simulink model "Chapter_4_Section_3_Model"  (R2017a)
settings: Solver=ode4  StartTime=0.0  StopTime=200  FixedStep=stp_sz  MaxStep=.0001  MinStep=.00005  RelTol=1e-7  AbsTol=1e-7  EnableMultiTasking=on
InitFcn:
  | load Chapter_4_Section_3
  | warning off
StopFcn:
  | save data.mat u_simulation v_simulation psi_simulation r_simulation npr_user_provided npr_achievable alpha_user_provided alpha_achievable stp_sz
  | clear all
  | load('data.mat')
  | delete('data.mat')
values from neighbouring files (symbols this model uses):
  A_disk = 13.2025431267    [Chapter_4_Section_3.mat]
  a_r11 = [-0.000865667853776 -0.901318756108 0.00874486630837 -0.00765974060328 0.00955717632387 0.00641813989061 -0.011076069832 0.00201248118094 -0.00501952733262 0.00315605586996 -0.00210851076531 0.0148609220099 ... (324 elements, 18x18)]    [Chapter_4_Section_3.mat]
  a_r13 = [-0.0294995912119 -4.91037219533 -0.00332739568397 0.0888755061346 -0.00681796875441 0.183812407485 0.0112008036726 0.10429312155 -0.0251601482875 -0.228675692165 0.00453476042855 0.0594697753606 ... (169 elements, 13x13)]    [Chapter_4_Section_3.mat]
  a_r15 = [-0.00127786555898 0.776225741104 -0.00474776997752 -0.00131066749835 0.0137520402687 -0.00211384579247 8.8019955143e-05 -0.00028996241197 -0.00129826872567 -0.0202543144732 0.0030370404199 -0.00453425604591 ... (169 elements, 13x13)]    [Chapter_4_Section_3.mat]
  a_r22 = [-0.000797108949019 -1.01015556887 0.00406573750109 -0.00111578544774 0.00423859757219 -0.00799128279013 0.00569024815652 -0.0167562674532 0.00334935655618 -0.000712432292804 0.00154242142086 0.00240437743229 ... (169 elements, 13x13)]    [Chapter_4_Section_3.mat]
  a_r24 = [-0.000686927823555 -0.95665602689 0.00244839898375 0.00145613314595 -0.00607023426216 0.0163996841317 0.00152022458075 -0.000736874734971 -0.00294919321651 -0.000761800577268 -0.00251686123035 -0.00197732815976 ... (169 elements, 13x13)]    [Chapter_4_Section_3.mat]
  a_r26 = [-0.194397873228 1.89810259721 -0.0873186628061 -0.241231729519 0.281206161775 -0.16994038615 -0.116565511469 -0.0496572593209 0.0216084469732 0.0912933167406 0.0299797727001 0.0314987707028 ... (169 elements, 13x13)]    [Chapter_4_Section_3.mat]
  a_r31 = [-0.00489112559449 -3.89960530455 -0.0361162658575 0.0265931197764 0.0034376033088 0.000316401308368 -0.0243996243526 0.0792200139858 -0.023187698537 -0.0726743997029 0.00400632061963 -0.0350516560041 ... (169 elements, 13x13)]    [Chapter_4_Section_3.mat]
  a_r33 = [-0.601431448276 0.50360246711 0.500115950342 -0.0452293844892 -0.0181314142185 -0.0323524621531 0.0355826051968 0.0329239610677 0.0940919952313 0.0566642992805 -0.0379178935102 0.0254835488846 ... (169 elements, 13x13)]    [Chapter_4_Section_3.mat]
  a_r35 = [-0.861988746714 -0.582511154549 0.34264856173 -0.0655310417272 -0.417167685168 0.183176698588 -0.473887691644 -0.225677727522 -0.133571139717 -0.218168843707 0.0850592077583 -0.0257492082836 ... (169 elements, 13x13)]    [Chapter_4_Section_3.mat]
  a_r42 = [-0.000411079312172 -0.966350953459 0.00419936729713 0.00358740198521 -0.00356571428733 -0.00958951498266 -0.00230062261745 -3.48708248632e-05 -0.00350313209064 -0.00772126326768 -0.0011918234528 -0.00149424537901 ... (169 elements, 13x13)]    [Chapter_4_Section_3.mat]
  a_r44 = [-0.000156115728087 -0.944139704333 -0.00242185567679 0.00620214191605 0.00232565005277 -0.00625050722164 0.00126021167241 -0.000681873506535 0.0011931592381 -0.00289361611357 -0.00138182415247 -0.00252837386868 ... (169 elements, 13x13)]    [Chapter_4_Section_3.mat]
  a_r46 = [-0.000218462457517 1.89677852742 0.00896242354968 -0.00290259500747 0.00225128874867 0.00254539590487 0.00120681433209 0.00261900930035 0.00149629742842 0.000796832004109 0.00199591847947 0.00352664402036 ... (169 elements, 13x13)]    [Chapter_4_Section_3.mat]
  a_r51 = [-0.0010898880101 0.776080724329 0.000225388678941 0.00375234840616 -0.00838297691459 -0.00447310416982 -0.0119510882322 -0.00692765468718 0.00227273345413 -0.0063592610709 0.000914007544175 0.00943534814934 ... (169 elements, 13x13)]    [Chapter_4_Section_3.mat]
  a_r53 = [-0.83377539904 0.569677058563 0.434285019976 0.157205409215 -0.397195569542 -0.255164078245 -0.141246880777 0.177451291189 -0.182828550566 0.0648162508754 0.244251292681 0.160100487197 ... (169 elements, 13x13)]    [Chapter_4_Section_3.mat]
  a_r55 = [-0.000352406331634 0.764343029796 0.00339830320259 -0.000678251137483 -0.00243783779313 -0.00215979913278 0.00196909451093 -0.00577428819561 -0.00349811892924 -0.00488920883323 0.00112064970343 0.000774855197444 ... (169 elements, 13x13)]    [Chapter_4_Section_3.mat]
  a_r62 = [-0.546519039316 -1.22303009993 0.393735845548 -0.120016588191 0.38151861373 -0.213578592342 -0.602267954372 -0.105716444149 -0.153151371839 -0.163939447448 -0.555540353196 0.0685401630267 ... (169 elements, 13x13)]    [Chapter_4_Section_3.mat]
  a_r64 = [-0.0406191100017 -5.18251105957 -0.115497941507 -0.0935821370219 0.180972853448 -0.0201998949456 -0.0698170640352 -0.0736823539521 -0.034828919888 0.0876659960431 -0.0419335596239 -0.0240984963396 ... (169 elements, 13x13)]    [Chapter_4_Section_3.mat]
  a_r66 = [-0.00276803466684 1.11530008029 0.0229779449181 0.0262185319857 0.00628472844795 0.000156167369042 -0.00250093023805 -0.0114435042874 -0.00826774415326 -0.00991601759993 -0.00812142854996 0.0148245002111 ... (169 elements, 13x13)]    [Chapter_4_Section_3.mat]
  A_rudder = 6    [Chapter_4_Section_3.mat]
  alpha_max = 0.392699081699    [Chapter_4_Section_3.mat]
  b_r11 = [-1.91804272115 -67.7547902158 12.3212653748 -6.25011871643 13.082442224 5.48501776184 -10.1596546398 2.56004852009 -4.74360113798 3.95981895348 -2.02856412397 18.3264246889 ... (18 elements, 18x1)]    [Chapter_4_Section_3.mat]
  b_r13 = [9.68113335046 8.54720242819 0.883931047444 -5.56576078332 1.72641800243 -13.8756826027 -2.702777864 -9.4621991361 5.92943514782 22.6516835054 -1.0074598861 -6.31102592982 ... (13 elements, 13x1)]    [Chapter_4_Section_3.mat]
  b_r22 = [-8.230214728 -263.156134326 24.2327808151 -4.87921448873 19.1715641288 -45.8768653263 26.6325387064 -91.9399975548 16.6663243552 -3.80929112747 7.68030110892 12.8381492859 ... (13 elements, 13x1)]    [Chapter_4_Section_3.mat]
  b_r24 = [20.6689502907 674.321335078 -41.3637763247 -19.2444203625 82.0775505272 -259.897803047 -22.2545830602 11.3827604156 43.2189922355 11.7516897475 36.9394390446 30.4503929007 ... (13 elements, 13x1)]    [Chapter_4_Section_3.mat]
  b_r26 = [206.794755218 -62.242559329 24.5666904254 184.158146246 -103.419961827 115.160111337 76.4499795128 20.3457431208 -13.1704465249 -41.5730935141 -18.1334448714 -14.4641153742 ... (13 elements, 13x1)]    [Chapter_4_Section_3.mat]
  b_r31 = [3.76230189948 5.16928151238 2.64945725635 -18.4251953385 -2.0625905672 -0.18887543415 4.20433084471 -14.07893046 13.0563354882 16.4007691754 -2.13849071942 8.28528512456 ... (13 elements, 13x1)]    [Chapter_4_Section_3.mat]
  b_r33 = [-425.265727934 16.4952177922 163.76327445 -15.539902078 -6.59006558263 -11.1862310226 12.8543123126 11.4260264426 33.8206936715 19.7626944669 -13.5783728882 8.91023495161 ... (13 elements, 13x1)]    [Chapter_4_Section_3.mat]
  b_r35 = [955.467057384 23.8174564739 -126.402446683 48.3788727465 168.435579445 -128.161344325 216.24493699 142.979450788 65.1193355403 134.911935543 -50.7648858119 13.1799100865 ... (13 elements, 13x1)]    [Chapter_4_Section_3.mat]
  b_r42 = [15.9360311823 665.959154186 -98.5777560157 -55.5400651809 61.9220987195 200.312325561 47.5124103398 0.631683490985 64.1219861023 155.750535985 22.3985447876 29.803792586 ... (13 elements, 13x1)]    [Chapter_4_Section_3.mat]
  b_r44 = [-27.1891200017 -1761.50772747 -283.391471232 367.311489951 182.522124626 -579.755911925 104.353356772 -62.2376848714 99.3185259533 -260.784153955 -116.536414334 -226.454300618 ... (13 elements, 13x1)]    [Chapter_4_Section_3.mat]
  b_r46 = [-26.6906838426 431.487773123 657.709356633 -144.976364483 114.646575538 180.775978583 85.0953284375 135.592940904 78.9082960716 55.2973047721 106.740201988 241.432567993 ... (13 elements, 13x1)]    [Chapter_4_Section_3.mat]
  b_r51 = [-27.9768378982 741.05041888 2.33758926296 57.3995096963 -127.005620965 -47.2947833409 -133.876425682 -98.5907202753 26.0445243962 -88.3721242204 10.7680008324 130.122749963 ... (13 elements, 13x1)]    [Chapter_4_Section_3.mat]
  b_r53 = [949.455593416 -23.2452293814 -157.318364745 -121.412853107 173.067821874 177.10214052 64.7164189373 -120.452255472 86.0623964314 -43.0643550932 -116.39314584 -105.497696438 ... (13 elements, 13x1)]    [Chapter_4_Section_3.mat]
  b_r55 = [-217.127382907 9506.32343029 1148.82922273 -188.742556573 -694.43970838 -709.996440288 566.872400877 -1877.38940059 -1026.37679575 -1566.80129668 332.089563592 247.692614281 ... (13 elements, 13x1)]    [Chapter_4_Section_3.mat]
  b_r62 = [259.61149635 16.5485296799 -38.0095496792 45.1883806678 -40.3107166739 78.3455844965 73.5107367495 37.0054960802 51.6709447748 22.7410486275 84.4875008959 -21.9559289205 ... (13 elements, 13x1)]    [Chapter_4_Section_3.mat]
  b_r64 = [156.539833252 187.686482031 376.820920142 59.4312894666 -548.902692032 17.0176436095 70.7484878223 206.821047291 37.1716677759 -243.032149857 114.824775027 27.0037475025 ... (13 elements, 13x1)]    [Chapter_4_Section_3.mat]
  b_r66 = [-314.266256408 5285.46587095 1093.01941502 1627.30071258 387.633965073 8.0986510694 -130.443621448 -701.343286032 -436.49966457 -600.0481003 -433.735518303 884.367320612 ... (13 elements, 13x1)]    [Chapter_4_Section_3.mat]
  bettas_CQ = [0 5.39 17.77 34.97 50.79 58.7 64.55 68.33 73.49 85.2 93.11 102.75 ... (40 elements, 1x40)]    [Chapter_4_Section_3.mat]    (also in looking_up_n.m = [0 5.39 17.77 34.97 50.79 58.7 64.55 68.33 73.49 85.2 93.11 )
  bettas_CT = [0 5.37 16.73 33.6 44.63 60.82 73.22 80.46 86.3 92.15 100.41 110.74 ... (52 elements, 1x52)]    [Chapter_4_Section_3.mat]    (also in looking_up_n.m = [0 5.37 16.73 33.6 44.63 60.82 73.22 80.46 86.3 92.15 100.41)
  c_r11 = [1.91804272142 -67.7547902158 -12.3212653748 -6.25011871643 -13.082442224 5.48501776185 -10.1596546398 -2.56004852009 -4.74360113798 -3.95981895348 -2.02856412396 -18.3264246889 ... (18 elements, 1x18)]    [Chapter_4_Section_3.mat]
  c_r13 = [9.68113335045 -8.54720242824 0.883931047418 5.56576078332 1.72641800244 13.8756826027 -2.702777864 9.4621991361 5.92943514781 -22.6516835054 -1.0074598861 6.31102592982 ... (13 elements, 1x13)]    [Chapter_4_Section_3.mat]
  c_r22 = [8.23021472807 -263.156134326 -24.2327808151 -4.87921448871 19.1715641288 45.8768653263 26.6325387064 91.9399975548 16.6663243552 3.80929112749 7.68030110892 -12.8381492859 ... (13 elements, 1x13)]    [Chapter_4_Section_3.mat]
  c_r24 = [20.6689502903 -674.321335078 -41.3637763247 19.2444203625 -82.0775505271 -259.897803047 22.2545830602 11.3827604156 -43.2189922355 11.7516897475 -36.9394390446 30.4503929007 ... (13 elements, 1x13)]    [Chapter_4_Section_3.mat]
  c_r26 = [-206.794755218 -62.2425593289 24.5666904254 -184.158146246 -103.419961827 -115.160111337 -76.4499795128 20.3457431209 13.1704465249 -41.5730935141 18.1334448714 -14.4641153742 ... (13 elements, 1x13)]    [Chapter_4_Section_3.mat]
  c_r31 = [3.76230189951 -5.16928151238 -2.64945725636 -18.4251953385 -2.0625905672 -0.188875434257 -4.2043308447 14.07893046 13.0563354882 -16.4007691754 -2.13849071943 -8.28528512456 ... (13 elements, 1x13)]    [Chapter_4_Section_3.mat]
  c_r33 = [-425.265727934 -16.4952177923 -163.76327445 15.539902078 -6.5900655826 11.1862310226 12.8543123126 -11.4260264426 33.8206936715 -19.7626944669 -13.5783728882 -8.91023495161 ... (13 elements, 1x13)]    [Chapter_4_Section_3.mat]
  c_r35 = [-955.467057384 23.8174564746 -126.402446683 -48.3788727464 168.435579445 128.161344325 216.24493699 -142.979450788 65.1193355403 -134.911935543 50.7648858119 13.1799100865 ... (13 elements, 1x13)]    [Chapter_4_Section_3.mat]
  c_r42 = [15.9360311824 -665.959154186 -98.5777560157 55.5400651809 -61.9220987195 200.312325561 47.5124103398 -0.631683490192 -64.1219861023 155.750535985 -22.3985447876 29.803792586 ... (13 elements, 1x13)]    [Chapter_4_Section_3.mat]
  c_r44 = [27.189120009 -1761.50772747 283.391471232 367.311489951 182.522124626 579.755911925 104.353356772 62.2376848713 99.3185259533 260.784153955 -116.536414334 226.454300618 ... (13 elements, 1x13)]    [Chapter_4_Section_3.mat]
  c_r46 = [26.6906838375 431.487773123 -657.709356633 -144.976364484 114.646575538 -180.775978583 -85.0953284373 135.592940904 78.9082960717 -55.297304772 106.740201988 -241.432567993 ... (13 elements, 1x13)]    [Chapter_4_Section_3.mat]
  c_r51 = [27.9768378982 741.05041888 2.33758926325 -57.3995096963 127.005620965 -47.2947833409 -133.876425682 98.5907202753 26.0445243962 88.3721242204 10.7680008324 -130.122749963 ... (13 elements, 1x13)]    [Chapter_4_Section_3.mat]
  c_r53 = [-949.455593416 -23.2452293814 -157.318364745 121.412853107 173.067821874 -177.10214052 64.7164189374 120.452255472 86.0623964314 43.0643550932 -116.39314584 105.497696438 ... (13 elements, 1x13)]    [Chapter_4_Section_3.mat]
  c_r55 = [217.12738291 9506.32343029 -1148.82922273 -188.742556576 -694.43970838 709.996440288 566.872400876 1877.38940059 -1026.37679575 1566.80129668 332.089563594 -247.69261428 ... (13 elements, 1x13)]    [Chapter_4_Section_3.mat]
  c_r62 = [-259.61149635 16.5485296799 -38.0095496792 -45.1883806678 -40.3107166739 -78.3455844965 73.5107367495 -37.0054960802 -51.6709447748 22.7410486275 84.4875008959 21.9559289205 ... (13 elements, 1x13)]    [Chapter_4_Section_3.mat]
  c_r64 = [-156.539833251 187.686482031 -376.820920142 59.4312894666 548.902692032 17.0176436097 70.7484878223 -206.82104729 37.1716677758 243.032149857 -114.824775027 27.0037475025 ... (13 elements, 1x13)]    [Chapter_4_Section_3.mat]
  c_r66 = [314.266256408 5285.46587095 1093.01941502 -1627.30071258 -387.633965073 8.09865107118 -130.443621448 701.343286032 -436.49966457 600.0481003 -433.735518303 -884.367320612 ... (13 elements, 1x13)]    [Chapter_4_Section_3.mat]
  CQs = [0.008 0.007 -0.002 -0.018 -0.037 -0.049 -0.06 -0.065 -0.068 -0.059 -0.057 -0.059 ... (40 elements, 1x40)]    [Chapter_4_Section_3.mat]    (also in looking_up_n.m = -0.1.*[-0.08 -0.07 0.02 0.18 0.37 0.49 0.6 0.65 0.68 0.59 0.)
  CTs = [0.32 0.29 0.19 0.01 -0.16 -0.46 -0.7 -0.77 -0.7 -0.63 -0.63 -0.69 ... (52 elements, 1x52)]    [Chapter_4_Section_3.mat]    (also in looking_up_n.m = [0.32 0.29 0.19 0.01 -0.16 -0.46 -0.7 -0.77 -0.7 -0.63 -0.63)
  d_r11 = 95.5285227708    [Chapter_4_Section_3.mat]
  d_r13 = -14.1628545989    [Chapter_4_Section_3.mat]
  d_r22 = 1468.51041279    [Chapter_4_Section_3.mat]
  d_r24 = -9785.77027698    [Chapter_4_Section_3.mat]
  d_r26 = -1700.92421833    [Chapter_4_Section_3.mat]
  d_r31 = -0.95522945761    [Chapter_4_Section_3.mat]
  d_r33 = 3827.81220596    [Chapter_4_Section_3.mat]
  d_r35 = -19539.5268707    [Chapter_4_Section_3.mat]
  d_r42 = -9418.04264727    [Chapter_4_Section_3.mat]
  d_r44 = 68252.1479072    [Chapter_4_Section_3.mat]
  d_r46 = -10162.1377852    [Chapter_4_Section_3.mat]
  d_r51 = 12054.4514237    [Chapter_4_Section_3.mat]
  d_r53 = -19539.5038011    [Chapter_4_Section_3.mat]
  d_r55 = 1991036.95813    [Chapter_4_Section_3.mat]
  d_r62 = -1405.47636444    [Chapter_4_Section_3.mat]
  d_r64 = -12342.2523681    [Chapter_4_Section_3.mat]
  d_r66 = 610786.440495    [Chapter_4_Section_3.mat]
  DEN = 5.34671106464e+28    [Chapter_4_Section_3.mat]
  dist_LOS = [-50 -49 -48 -47 -46 -45 -44 -43 -42 -41 -40 -39 ... (1051 elements, 1x1051)]    [Chapter_4_Section_3.mat]
  Dpr = 4.1    [Chapter_4_Section_3.mat]    (also in looking_up_n.m = u(4))
  Dw = 0.110526315789    [Chapter_4_Section_3.mat]
  dx = 10    [Chapter_4_Section_3.mat]
  dxr = 48.75    [Chapter_4_Section_3.mat]
  dy = 2    [Chapter_4_Section_3.mat]
  dz = 0.8    [Chapter_4_Section_3.mat]
  dzr = 0.514285714286    [Chapter_4_Section_3.mat]
  g = 10    [Chapter_4_Section_3.mat]
  gravity = 10    [Chapter_4_Section_3.mat]
  INDEX = [1 2 3 4 5 6 7 8 9]    [Chapter_4_Section_3.mat]
  Ix = 724554000    [Chapter_4_Section_3.mat]
  Iy = 4528460000    [Chapter_4_Section_3.mat]
  Iz = 4528460000    [Chapter_4_Section_3.mat]
  k_wave = [0.0157865285852 0.0224311321394 0.0345394916241 0.0578593033576 0.0778685019714 0.0983501894009 0.10403521245 0.134043066308 0.155236404606 0.203205074918 0.220032771713 0.262178651673 ... (20 elements, 1x20)]    [Chapter_4_Section_3.mat]
  Last_Pt_Accuracy = 30    [Chapter_4_Section_3.mat]
  LBP = 100    [Chapter_4_Section_3.mat]
  m = 7264000    [Chapter_4_Section_3.mat]
  phase = [4.61787442739 6.09845039199 5.44708367148 0.54182753101 2.30238916367 2.31974450279 4.30416083443 3.75697809799 4.95971993271 2.31003141527 1.29451121971 0.54454197722 ... (20 elements, 1x20)]    [Chapter_4_Section_3.mat]
  phi_0 = 0    [Chapter_4_Section_3.mat]
  psi_0 = 0    [Chapter_4_Section_3.mat]
  R_convrg = 220    [Chapter_4_Section_3.mat]
  radius_LOS = [166.575605377 166.637026665 166.698699321 166.760625342 166.82280675 166.885245588 166.947943925 167.010903854 167.074127493 167.137616985 167.201374499 167.265402228 ... (1051 elements, 1x1051)]    [Chapter_4_Section_3.mat]
  raw = 1000    [Chapter_4_Section_3.mat]    (also in looking_up_n.m = u(3))
  s = 0.15    [Chapter_4_Section_3.mat]
  S11 = 5.22457985714e+28    [Chapter_4_Section_3.mat]
  S13 = 3.79917831589e+26    [Chapter_4_Section_3.mat]
  S15 = -4.97006200608e+19    [Chapter_4_Section_3.mat]
  S22 = 4.58630932583e+28    [Chapter_4_Section_3.mat]
  S24 = 9.38800137353e+19    [Chapter_4_Section_3.mat]
  S26 = 1.30387886946e+18    [Chapter_4_Section_3.mat]
  S31 = 3.83422033136e+26    [Chapter_4_Section_3.mat]
  S33 = 1.77296018417e+28    [Chapter_4_Section_3.mat]
  S35 = 2.44593333777e+19    [Chapter_4_Section_3.mat]
  S42 = 8.93369784557e+19    [Chapter_4_Section_3.mat]
  S44 = 7.37931315974e+19    [Chapter_4_Section_3.mat]
  S46 = 27990784014.6    [Chapter_4_Section_3.mat]
  S51 = -4.98658939538e+19    [Chapter_4_Section_3.mat]
  S53 = 2.45188465874e+19    [Chapter_4_Section_3.mat]
  S55 = 1.18069051188e+19    [Chapter_4_Section_3.mat]
  S62 = 1.30580221388e+18    [Chapter_4_Section_3.mat]
  S64 = 23535167243.9    [Chapter_4_Section_3.mat]
  S66 = 1.18069078235e+19    [Chapter_4_Section_3.mat]
  ... (+18 more)
undefined symbols (not defined in the file or in its folder): magnitude
libraries: simulink x9
(part 1 of 6)
CloseFcn:
  | rtwprivate ssgencode ModelCloseRequest editted_june25_edit_radius
settings Model: Creator=Nassim Khaled  LastModifiedBy=nassi
settings SolverCC: MaxConsecutiveMinStep=100
settings DataIOCC: Decimation=100  LimitDataPoints=on  MaxDataPoints=2500000  SaveFormat=Array  SignalLoggingSaveFormat=ModelDataLogs  SaveOutput=off  SignalLogging=off  SaveTime=off  OutputOption=SpecifiedOutputTimes  OutputTimes=0:.2:200
settings OptimizationCC: BooleanDataType=off  OptimizeBlockIOStorage=off  BufferReuse=off  GlobalBufferReuse=off  ExpressionFolding=off  ExpressionDepthLimit=2147483647  LocalBlockOutputs=off  InitFltsAndDblsToZero=on  LifeSpan=inf
settings DebuggingCC: ConsistencyChecking=warning  SaveWithParameterizedLinksMsg=none  UnderspecifiedInitializationDetection=Classic  MergeDetectMultiDrivingBlocksExec=none  SignalResolutionControl=TryResolveAllWithWarning  MaxConsecutiveZCsMsg=warning  SolverPrmCheckMsg=warning  MultiTaskDSMMsg=warning  MultiTaskCondExecSysMsg=warning  MultiTaskRateTransMsg=warning  FcnCallInpInsideContextMsg=warning  ModelReferenceExtraNoncontSigs=warning  StateNameClashWarn=warning  SFUnexpectedBacktrackingDiag=warning  SFNoUnconditionalDefaultTransitionDiag=warning  SFExecutionAtInitializationDiag=none
settings HardwareCC: ProdBitPerPointer=32  ProdBitPerSizeT=32  ProdBitPerPtrDiffT=32  ProdLargestAtomicFloat=None  ProdIntDivRoundTo=Undefined  ProdEndianess=Unspecified  ProdWordSize=32  ProdHWDeviceType=32-bit Generic  TargetBitPerPointer=64  TargetBitPerSizeT=64  TargetBitPerPtrDiffT=64  TargetLongLongMode=on  TargetIntDivRoundTo=Zero  TargetEndianess=LittleEndian  TargetWordSize=64  TargetHWDeviceType=MATLAB Host  ProdEqTarget=off
settings ModelReferenceCC: PropagateSignalLabelsOutOfModel=off
settings SFSimCC: SimParseCustomCode=off
settings RTWCC: SystemTargetFile=rsim.tlc  TemplateMakefile=rsim_default_tmf  Description=Rapid Simulation Target
settings ConfigComp: CovMetricSettings=dw  CovHtmlReporting=on  CovSaveCumulativeToWorkspaceVar=on  CovSaveSingleToWorkspaceVar=on  CovExternalEMLEnable=off

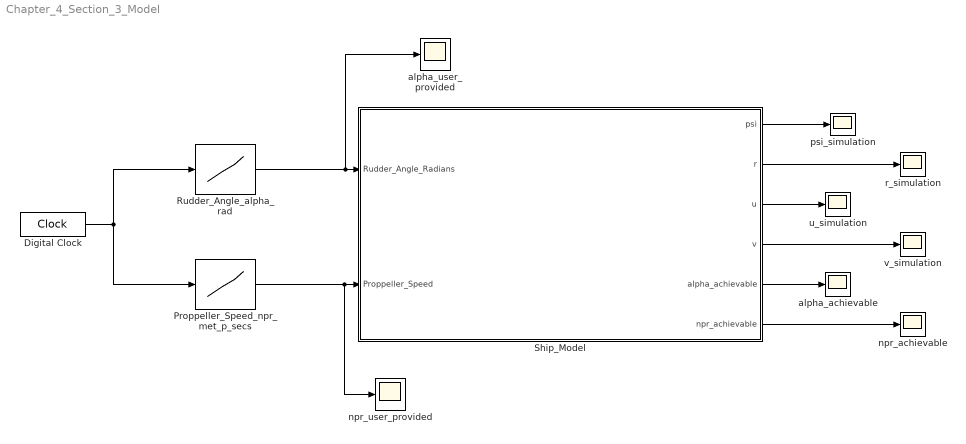
== system Chapter_4_Section_3_Model ==
  Digital Clock : DigitalClock  SampleTime=stp_sz
  Proppeller_Speed_npr_met_p_secs : Lookup_n-D  NumberOfTableDimensions=1  BreakpointsForDimension1=[0 75 100.2 150]  Table=[10 10 15 15 ]  InternalRulePriority=Speed  RndMeth=Simplest  InputSameDT=on
  Rudder_Angle_alpha_rad : Lookup_n-D  NumberOfTableDimensions=1  BreakpointsForDimension1="[0 25  42.5 150]"  Table=[0 0 0.1745 0.1745]  InternalRulePriority=Speed  RndMeth=Simplest  InputSameDT=on
  Ship_Model : Subsystem
  alpha_achievable : Scope
  alpha_user_provided : Scope
  npr_achievable : Scope
  npr_user_provided : Scope
  psi_simulation : Scope
  r_simulation : Scope
  u_simulation : Scope
  v_simulation : Scope
  wires:
  Proppeller_Speed_npr_met_p_secs/1 -> Ship_Model/2(Proppeller_Speed), npr_user_provided/1
  Rudder_Angle_alpha_rad/1 -> alpha_user_provided/1, Ship_Model/1(Rudder_Angle_Radians)
  Ship_Model/1(psi) -> psi_simulation/1
  Ship_Model/2(r) -> r_simulation/1
  Ship_Model/3(u) -> u_simulation/1
  Ship_Model/4(v) -> v_simulation/1
  Digital Clock/1 -> Rudder_Angle_alpha_rad/1, Proppeller_Speed_npr_met_p_secs/1
  Ship_Model/5(alpha_achievable) -> alpha_achievable/1
  Ship_Model/6(npr_achievable) -> npr_achievable/1

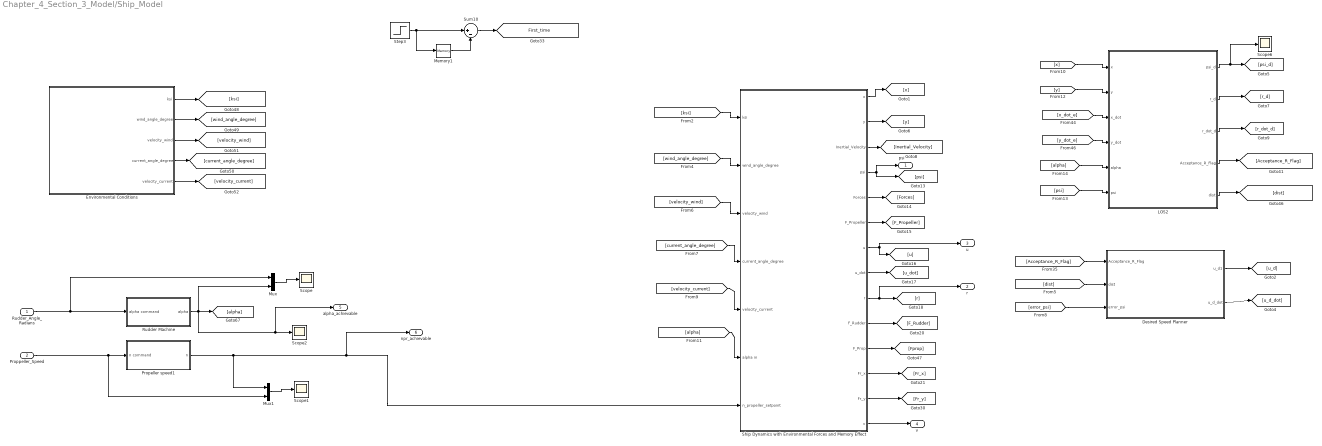
== system Chapter_4_Section_3_Model/Ship_Model ==
  Rudder_Angle_Radians : Inport
  Proppeller_Speed : Inport  Port=2
  Desired Speed Planner : Subsystem
  Environmental Conditions : Subsystem
  LOS2 : Subsystem
  Memory1 : Memory  InheritSampleTime=on
  Mux : Mux  Inputs=2
  Mux1 : Mux  Inputs=2
  Propeller speed1 : Subsystem
  Rudder Machine : Subsystem
  Scope{,1..2,6} (4 alike) : Scope
  Ship Dynamics with Environmental Forces and Memory Effect : Subsystem
  Step3 : Step  Time=0  SampleTime=0
  Sum10 : Sum  Inputs=|+-
  psi : Outport
  r : Outport  Port=2
  u : Outport  Port=3
  v : Outport  Port=4
  alpha_achievable : Outport  Port=5
  npr_achievable : Outport  Port=6
  tag scope: First_time=global
  wires:
  Step3/1 -> Memory1/1, Sum10/1
  [dist] -> Desired Speed Planner/2(dist)
  [y_dot_e] -> LOS2/4(y_dot)
  [alpha] -> LOS2/5(alpha)
  [current_angle_degree] -> Ship Dynamics with Environmental Forces and Memory Effect/4(current_angle_degree)
  [alpha] -> Ship Dynamics with Environmental Forces and Memory Effect/6(alpha in)
  [wind_angle_degree] -> Ship Dynamics with Environmental Forces and Memory Effect/2(wind_angle_degree)
  [x_dot_e] -> LOS2/3(x_dot)
  LOS2/1(psi_d) -> Scope6/1, [psi_d]
  [psi] -> LOS2/6(psi)
  Environmental Conditions/3(velocity_wind) -> [velocity_wind]
  [velocity_wind] -> Ship Dynamics with Environmental Forces and Memory Effect/3(velocity_wind)
  Memory1/1 -> Sum10/2
  [error_psi] -> Desired Speed Planner/3(error_psi)
  Environmental Conditions/1(ksi) -> [ksi]
  Environmental Conditions/2(wind_angle_degree) -> [wind_angle_degree]
  [x] -> LOS2/1(x)
  [ksi] -> Ship Dynamics with Environmental Forces and Memory Effect/1(ksi)
  [y] -> LOS2/2(y)
  LOS2/2(r_d) -> [r_d]
  [Acceptance_R_Flag] -> Desired Speed Planner/1(Acceptance_R_Flag)
  [velocity_current] -> Ship Dynamics with Environmental Forces and Memory Effect/5(velocity_current)
  Sum10/1 -> [First_time]
  Environmental Conditions/5(velocity_current) -> [velocity_current]
  Environmental Conditions/4(current_angle_degree) -> [current_angle_degree]
  Ship Dynamics with Environmental Forces and Memory Effect/2(y) -> [y]
  Ship Dynamics with Environmental Forces and Memory Effect/8(u_dot) -> [u_dot]
  Ship Dynamics with Environmental Forces and Memory Effect/5(Forces) -> [Forces]
  LOS2/3(r_dot_d) -> [r_dot_d]
  Desired Speed Planner/1(u_d1) -> [u_d]
  Ship Dynamics with Environmental Forces and Memory Effect/1(x) -> [x]
  Ship Dynamics with Environmental Forces and Memory Effect/13(Fr_y) -> [Fr_y]
  Proppeller_Speed/1 -> Propeller speed1/1(n command), Mux1/2
  Ship Dynamics with Environmental Forces and Memory Effect/4(psi) -> psi/1, [psi]
  Ship Dynamics with Environmental Forces and Memory Effect/9(r) -> r/1, [r]
  Desired Speed Planner/2(u_d_dot) -> [u_d_dot]
  Ship Dynamics with Environmental Forces and Memory Effect/6(F_Propeller) -> [F_Propeller]
  Ship Dynamics with Environmental Forces and Memory Effect/11(F_Prop) -> [Fprop]
  Mux/1 -> Scope/1
  Ship Dynamics with Environmental Forces and Memory Effect/7(u) -> u/1, [u]
  LOS2/4(Acceptance_R_Flag) -> [Acceptance_R_Flag]
  LOS2/5(dist) -> [dist]
  Ship Dynamics with Environmental Forces and Memory Effect/10(F_Rudder) -> [F_Rudder]
  Ship Dynamics with Environmental Forces and Memory Effect/3(Inertial_Velocity) -> [Inertial_Velocity]
  Ship Dynamics with Environmental Forces and Memory Effect/12(Fr_x) -> [Fr_x]
  Rudder_Angle_Radians/1 -> Rudder Machine/1(alpha command), Mux/1
  Rudder Machine/1(alpha) -> alpha_achievable/1, Scope2/1, Mux/2, [alpha]
  Propeller speed1/1(n) -> Mux1/1, npr_achievable/1, Ship Dynamics with Environmental Forces and Memory Effect/7(n_propeller_setpoint)
  Mux1/1 -> Scope1/1
  Ship Dynamics with Environmental Forces and Memory Effect/14(v) -> v/1

== system Chapter_4_Section_3_Model/Ship_Model/Desired Speed Planner ==
  Acceptance_R_Flag : Inport
  dist : Inport  Port=2
  error_psi : Inport  Port=3
  Abs : Abs
  Derivative2 : Derivative
  If : If  NumInputs=2  IfExpression=u1 > 3 & u2<0.05
  If Action Subsystem : Subsystem  TreatAsAtomicUnit=on
  If Action Subsystem1 : Subsystem  TreatAsAtomicUnit=on
  Logical Operator : Logic  Operator=NOT  AllPortsSameDT=off
  Memory : Memory  X0=6
  Memory13 : Memory  X0=6
  Merge1 : Merge  InitialOutput=1
  Product : Product  RndMeth=Zero
  Saturation : Saturate  UpperLimit=6  LowerLimit=6
  Scope6 : Scope
  u_d1 : Outport
  u_d_dot : Outport  Port=2
  wires:
  If/1 -> If Action Subsystem/Action
  Abs/1 -> If/2
  Memory/1 -> If Action Subsystem/1(In1)
  If/2 -> If Action Subsystem1/Action
  [u_d] -> Memory13/1
  Memory13/1 -> If Action Subsystem1/1(In1)
  If Action Subsystem/1(Out1) -> Merge1/1
  If Action Subsystem1/1(Out1) -> Merge1/2
  Merge1/1 -> Saturation/1
  Saturation/1 -> u_d1/1, Derivative2/1, Scope6/1, [u_d]
  Logical Operator/1 -> Product/1
  Product/1 -> If/1
  Acceptance_R_Flag/1 -> Logical Operator/1
  dist/1 -> Product/2
  error_psi/1 -> Abs/1
  Derivative2/1 -> u_d_dot/1
  [u_d] -> Memory/1

== system Chapter_4_Section_3_Model/Ship_Model/Environmental Conditions ==
  Constant : Constant
  Constant{1..3,6..10} (8 alike) : Constant  Value=0
  Constant4 : Constant  Value=5
  Constant5 : Constant
  Demux : Demux  Outputs=5
  Mux : Mux  Inputs=5
  Mux1 : Mux  Inputs=5
  Switch : Switch  Criteria=u2 > Threshold
  ksi : Outport
  wind_angle_degree : Outport  Port=2
  velocity_wind : Outport  Port=3
  current_angle_degree : Outport  Port=4
  velocity_current : Outport  Port=5
  wires:
  Constant/1 -> Switch/2
  Constant1/1 -> Mux/1
  Constant2/1 -> Mux/2
  Constant4/1 -> Mux/3
  Constant3/1 -> Mux/4
  Constant5/1 -> Mux/5
  Mux/1 -> Switch/1
  Constant6/1 -> Mux1/1
  Constant7/1 -> Mux1/2
  Constant9/1 -> Mux1/3
  Constant8/1 -> Mux1/4
  Constant10/1 -> Mux1/5
  Mux1/1 -> Switch/3
  Switch/1 -> Demux/1
  Demux/1 -> ksi/1
  Demux/2 -> wind_angle_degree/1
  Demux/3 -> velocity_wind/1
  Demux/4 -> current_angle_degree/1
  Demux/5 -> velocity_current/1

== system Chapter_4_Section_3_Model/Ship_Model/LOS2 ==
  note: i am minimizing the abrupt change in the angle psi_d
      | when there is a shift to the next way point
  note: angle of the rudder
  note: heading of the ship
  x : Inport
  y : Inport  Port=2
  x_dot : Inport  Port=3
  y_dot : Inport  Port=4
  alpha : Inport  Port=5
  psi : Inport  Port=6
  Breivik Model for psi : Subsystem
  Memory4 : Memory  X0=1  InheritSampleTime=on
  Subsystem1 : Subsystem
  psi_d : Outport
  r_d : Outport  Port=2
  r_dot_d : Outport  Port=3
  Acceptance_R_Flag : Outport  Port=4
  dist : Outport  Port=5
  wires:
  [index] -> Memory4/1
  Memory4/1 -> Subsystem1/3(index_i)
  [x] -> Subsystem1/1(x)
  [y] -> Subsystem1/2(y)
  x/1 -> [x]
  y/1 -> [y]
  x_dot/1 -> [x_dot]
  y_dot/1 -> [y_dot]
  [x_dot] -> Subsystem1/4(x_dot)
  [y_dot] -> Subsystem1/5(y_dot)
  Subsystem1/1(index_i_update) -> [index]
  Subsystem1/2(x_los) -> [x_los]
  Subsystem1/3(y_los) -> [y_los]
  Subsystem1/4(dist) -> dist/1
  [x] -> Breivik Model for psi/1(x)
  [y] -> Breivik Model for psi/2(y)
  [x_los] -> Breivik Model for psi/3(x_los)
  [y_los] -> Breivik Model for psi/4(y_los)
  Breivik Model for psi/1(psi_d) -> psi_d/1
  Breivik Model for psi/2("psi_dot ") -> r_d/1
  Breivik Model for psi/3(psi_dot_dot) -> r_dot_d/1
  alpha/1 -> [alpha]
  psi/1 -> [psi]
  [alpha] -> Subsystem1/6(alpha)
  [psi] -> Subsystem1/7(psi)
  Subsystem1/5(Acceptance_R_Flag) -> Acceptance_R_Flag/1

== system Chapter_4_Section_3_Model/Ship_Model/Propeller speed1 ==
  n command : Inport
  Rate Limiter : RateLimiter  RisingSlewLimit=0.2  FallingSlewLimit=-0.2  SampleTimeMode=inherited  InitialCondition=10
  Saturation : Saturate  UpperLimit=30  LowerLimit=0.1
  n : Outport
  wires:
  Saturation/1 -> Rate Limiter/1
  n command/1 -> Saturation/1
  Rate Limiter/1 -> n/1

== system Chapter_4_Section_3_Model/Ship_Model/Rudder Machine ==
  alpha command : Inport
  Rate Limiter : RateLimiter  RisingSlewLimit=0.01  FallingSlewLimit=-0.01  SampleTimeMode=inherited
  Saturation : Saturate  UpperLimit=alpha_max  LowerLimit=-alpha_max
  alpha : Outport
  wires:
  alpha command/1 -> Saturation/1
  Saturation/1 -> Rate Limiter/1
  Rate Limiter/1 -> alpha/1

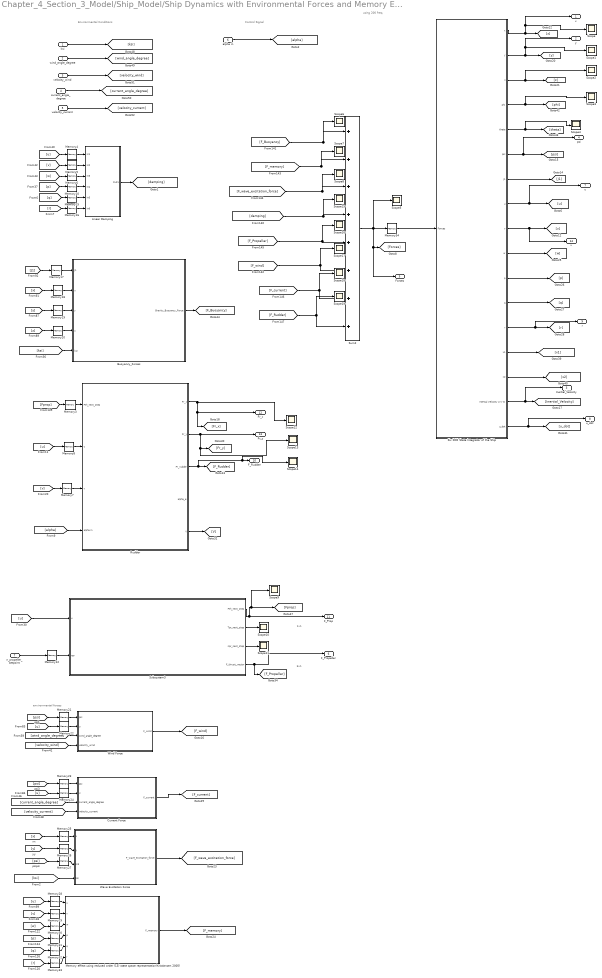
== system Chapter_4_Section_3_Model/Ship_Model/Ship Dynamics with Environmental Forces and Memory Effect ==
  note: using 200 freq.
  note: environmental forces
  note: Environmental Conditions
  note: Control Signal
  note: 1x1
  note: 6x1
  ksi : Inport
  wind_angle_degree : Inport  Port=2
  velocity_wind : Inport  Port=3
  current_angle_degree : Inport  Port=4
  velocity_current : Inport  Port=5
  alpha in : Inport  Port=6
  n_propeller_setpoint : Inport  Port=7
  Buoyancy_Forces : Subsystem
  Current Force : Subsystem
  Linear Damping : Subsystem
  Memory effect using reduced order (13) state space representation(Kristiansen 2005) : Subsystem
  Memory{4..8,10,15..16,18..33} (24 alike) : Memory  InheritSampleTime=on
  Memory12 : Memory  X0=10  InheritSampleTime=on
  Memory17 : Memory  X0=[1 0 0;0 1 0; 0 0 1]  InheritSampleTime=on
  Memory3 : Memory  X0=6  InheritSampleTime=on
  Memory34 : Memory  X0=[0;0;0;0;0;0]  InheritSampleTime=on
  Rudder : Subsystem
  Scope{,1..19} (20 alike) : Scope
  Six DOF State Integrator of the Ship : Subsystem
  Subsystem3 : Subsystem
      mask Display: image(imread('propeller.jpg'))
  Sum2 : Sum  Inputs=|+|+|+|+|+|+|+|+|
  Wave Excitation Force : Subsystem
  Wind Force : Subsystem
  x : Outport
  y : Outport  Port=2
  Inertial_Velocity : Outport  Port=3
  psi : Outport  Port=4
  Forces : Outport  Port=5
  F_Propeller : Outport  Port=6
  u : Outport  Port=7
  u_dot : Outport  Port=8
  r : Outport  Port=9
  F_Rudder : Outport  Port=10
  F_Prop : Outport  Port=11
  Fr_x : Outport  Port=12
  Fr_y : Outport  Port=13
  v : Outport  Port=14
  wires:
  Sum2/1 -> Scope5/1, Memory34/1, [Forces], Forces/1
  [u] -> Memory8/1
  [v] -> Memory7/1
  Rudder/1(Fr_x) -> [Fr_x], Fr_x/1, Scope12/1
  Rudder/2(Fr_y) -> Scope13/1, [Fr_y], Fr_y/1
  Memory7/1 -> Rudder/3(v)
  Rudder/5(V) -> [V]
  Memory8/1 -> Rudder/2(u)
  [Fprop] -> Memory3/1
  [J1] -> Memory17/1
  [x] -> Memory18/1
  Buoyancy_Forces/1(Gravity_Buoyancy_Force) -> [F_Buoyancy]
  [y] -> Memory19/1
  [z] -> Memory20/1
  [psi] -> Memory21/1
  [u] -> Memory22/1
  [psi] -> Memory23/1
  [u] -> Memory24/1
  [psi] -> Memory27/1
  [x] -> Memory25/1
  [y] -> Memory26/1
  Memory effect using reduced order (13) state space representation(Kristiansen 2005)/1(F_memory) -> [F_memory]
  [u] -> Memory28/1
  [v] -> Memory29/1
  [w] -> Memory30/1
  [p] -> Memory31/1
  [q] -> Memory32/1
  [r] -> Memory33/1
  [F_Buoyancy] -> Scope6/1, Sum2/1
  [F_memory] -> Scope7/1, Sum2/2
  [F_wave_excitation_force] -> Scope8/1, Sum2/3
  [damping] -> Scope15/1, Sum2/4
  [F_Propeller] -> Scope16/1, Sum2/5
  [F_wind] -> Scope17/1, Sum2/6
  [F_current] -> Scope18/1, Sum2/7
  [F_Rudder] -> Scope19/1, Sum2/8
  Linear Damping/1(Out1) -> [damping]
  [u] -> Memory4/1
  [v] -> Memory5/1
  [w] -> Memory6/1
  [p] -> Memory10/1
  [q] -> Memory15/1
  [r] -> Memory16/1
  Memory4/1 -> Linear Damping/1(In1)
  Memory5/1 -> Linear Damping/2(In2)
  Memory6/1 -> Linear Damping/3(In3)
  Memory10/1 -> Linear Damping/4(In4)
  Memory15/1 -> Linear Damping/5(In5)
  Memory16/1 -> Linear Damping/6(In6)
  Memory3/1 -> Rudder/1(Fth_next_step)
  Memory17/1 -> Buoyancy_Forces/1(J1)
  Memory18/1 -> Buoyancy_Forces/2(x)
  Memory19/1 -> Buoyancy_Forces/3(y)
  Memory20/1 -> Buoyancy_Forces/4(z)
  Memory21/1 -> Wind Force/1(psi)
  Memory22/1 -> Wind Force/2(u)
  Memory23/1 -> Current Force/1(psi)
  Memory24/1 -> Current Force/2(u)
  Memory25/1 -> Wave Excitation Force/1(x)
  Memory26/1 -> Wave Excitation Force/2(y)
  Memory27/1 -> Wave Excitation Force/3(In3)
  Memory28/1 -> Memory effect using reduced order (13) state space representation(Kristiansen 2005)/1(u)
  Memory29/1 -> Memory effect using reduced order (13) state space representation(Kristiansen 2005)/2(v)
  Memory30/1 -> Memory effect using reduced order (13) state space representation(Kristiansen 2005)/3(w)
  Memory31/1 -> Memory effect using reduced order (13) state space representation(Kristiansen 2005)/4(p)
  Memory32/1 -> Memory effect using reduced order (13) state space representation(Kristiansen 2005)/5(q)
  Memory33/1 -> Memory effect using reduced order (13) state space representation(Kristiansen 2005)/6(r)
  Memory34/1 -> Six DOF State Integrator of the Ship/1(Forces)
  [alpha] -> Rudder/4(alpha in)
  [ksi] -> Buoyancy_Forces/5(ksi)
  [wind_angle_degree] -> Wind Force/3(wind_angle_degree)
  [velocity_wind] -> Wind Force/4(velocity_wind)
  [current_angle_degree] -> Current Force/3(current_angle_degree)
  [velocity_current] -> Current Force/4(velocity_current)
  [ksi] -> Wave Excitation Force/4(ksi)
  ksi/1 -> [ksi]
  wind_angle_degree/1 -> [wind_angle_degree]
  velocity_wind/1 -> [velocity_wind]
  current_angle_degree/1 -> [current_angle_degree]
  velocity_current/1 -> [velocity_current]
  alpha in/1 -> [alpha]
  Six DOF State Integrator of the Ship/1(x) -> [x], Scope/1, x/1
  Six DOF State Integrator of the Ship/2(y) -> [y], Scope1/1, y/1
  Six DOF State Integrator of the Ship/3(z) -> Scope2/1, [z]
  Six DOF State Integrator of the Ship/4(phi) -> Scope3/1, [phi]
  Six DOF State Integrator of the Ship/5(theta) -> Scope4/1, [theta]
  Six DOF State Integrator of the Ship/6(psi) -> [psi], psi/1
  Six DOF State Integrator of the Ship/7(J1) -> [J1]
  Six DOF State Integrator of the Ship/8(u) -> u/1, [u]
  Six DOF State Integrator of the Ship/9(v) -> v/1, [v]
  Six DOF State Integrator of the Ship/10(w) -> [w]
  Six DOF State Integrator of the Ship/11(p) -> [p]
  Six DOF State Integrator of the Ship/12(q) -> [q]
  Six DOF State Integrator of the Ship/13(r) -> [r], r/1
  Six DOF State Integrator of the Ship/14(x1) -> [x1]
  Six DOF State Integrator of the Ship/15(x2) -> [x2]
  Six DOF State Integrator of the Ship/16(Inertial Velcoity U V W) -> [Inertial_Velocity], Inertial_Velocity/1
  Six DOF State Integrator of the Ship/17(u_dot) -> [u_dot], u_dot/1
  Rudder/3(Fr_rudder) -> [F_Rudder], Scope14/1, F_Rudder/1
  [u] -> Subsystem3/1(u)
  Memory12/1 -> Subsystem3/2(npr)
  Subsystem3/1(Fth_next_step) -> F_Prop/1, Scope9/1, [Fprop]
  Subsystem3/2(Tpr_next_step) -> Scope10/1
  Subsystem3/3(npr_next_step) -> Scope11/1
  Subsystem3/4(F_thrust_vector) -> F_Propeller/1, [F_Propeller]
  n_propeller_setpoint/1 -> Memory12/1
  Wind Force/1(F_wind) -> [F_wind]
  Current Force/1(F_current) -> [F_current]
  Wave Excitation Force/1(F_wave_excitation_force) -> [F_wave_excitation_force]

== system Chapter_4_Section_3_Model/Ship_Model/Desired Speed Planner/If Action Subsystem ==
  In1 : Inport
  Action Port : ActionPort  PropagateVarSize=During execution  ActionType=then
  Sum : Sum  Inputs=|+-
  deceleration slope : Constant  Value=0.01/30
  Out1 : Outport
  wires:
  In1/1 -> Sum/1
  deceleration slope/1 -> Sum/2
  Sum/1 -> Out1/1

== system Chapter_4_Section_3_Model/Ship_Model/Desired Speed Planner/If Action Subsystem1 ==
  In1 : Inport
  Action Port : ActionPort  PropagateVarSize=During execution  ActionType=else
  Sum : Sum  Inputs=|++
  deceleration slope : Constant  Value=0.01/30
  Out1 : Outport
  wires:
  Sum/1 -> Out1/1
  deceleration slope/1 -> Sum/2
  In1/1 -> Sum/1

== system Chapter_4_Section_3_Model/Ship_Model/LOS2/Breivik Model for psi ==
  x : Inport
  y : Inport  Port=2
  x_los : Inport  Port=3
  y_los : Inport  Port=4
  Add : Sum  Inputs=+-
  Add1 : Sum  Inputs=+-
  Heading Angle Filter : Subsystem
  Memory1 : Memory  InheritSampleTime=on
  Memory2 : Memory  InheritSampleTime=on
  Memory3 : Memory  InheritSampleTime=on
  Subsystem2 : Subsystem
  Trigonometric Function : Trigonometry  Operator=atan2
  pi2inf : MATLAB Function  TreatAsAtomicUnit=on
  psi_d1 : Subsystem
  psi_d : Outport
  "psi_dot " : Outport  Port=2
  psi_dot_dot : Outport  Port=3
  wires:
  [y_los] -> Add/1
  [y] -> Add/2
  [x_los] -> Add1/1
  [x] -> Add1/2
  Add/1 -> Trigonometric Function/1
  Add1/1 -> Trigonometric Function/2
  Trigonometric Function/1 -> [psi_d]
  [x_los] -> pi2inf/1(x_los)
  [y_los] -> pi2inf/2(y_los)
  [x] -> pi2inf/3(x)
  [y] -> pi2inf/4(y)
  [state_k] -> Memory1/1
  Memory2/1 -> pi2inf/6(psi_k_1)
  [psi_d] -> pi2inf/7(psi_k)
  [accumulation] -> Memory3/1
  Memory1/1 -> pi2inf/5(state_k_1)
  [psi_d] -> Memory2/1
  Memory3/1 -> pi2inf/8(accumulation_k_1)
  [accumulation] -> Heading Angle Filter/1(In1)
  Heading Angle Filter/1(psi) -> Subsystem2/1(x [-inf inf])
  Subsystem2/1(y [-pi pi]) -> psi_d1/1(psi [-pi pi])
  x/1 -> [x]
  y/1 -> [y]
  x_los/1 -> [x_los]
  y_los/1 -> [y_los]
  psi_d1/1(psi [0 2pi]) -> psi_d/1
  Heading Angle Filter/2(psi_dot) -> "psi_dot "/1
  Heading Angle Filter/3(psi_dot_dot) -> psi_dot_dot/1
  pi2inf/1(state_k) -> [state_k]
  pi2inf/2(accumulation_k) -> [accumulation]

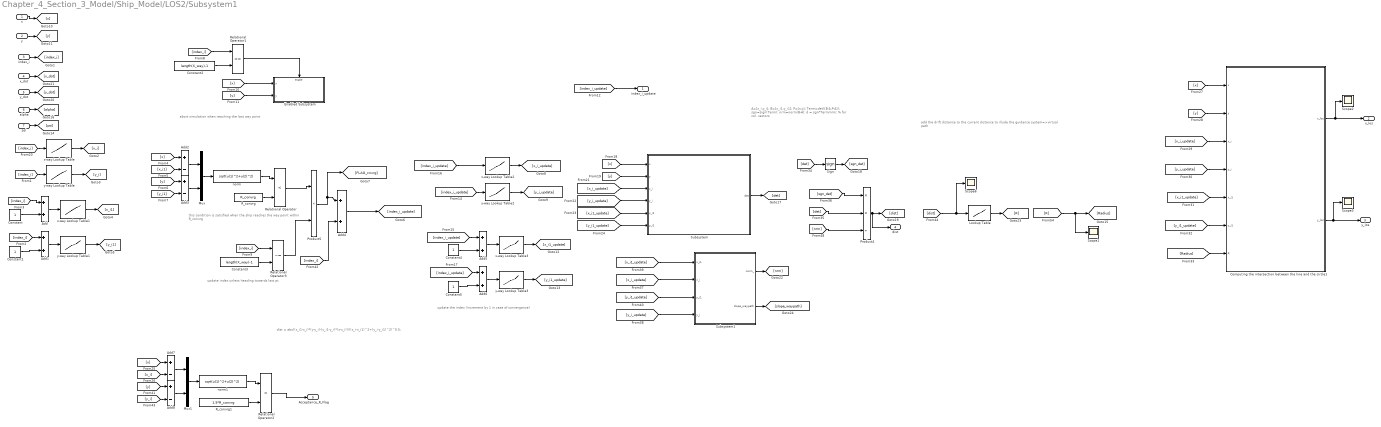
== system Chapter_4_Section_3_Model/Ship_Model/LOS2/Subsystem1 ==
  note: this condition is satisfied when the ship
      | reaches the way point within R_convrg
  note: abort simulation when reaching the last way point
  note: update the index (increment by 1 in case of convergance)
  note: dist = abs((x_i1-x_i)*(y-y_i)-(y_i1-y_i)*(x-x_i))/((x_i-x_i1)^2+(y_i-y_i1)^2)^0.5;
  note: A=[x_i;y_i];
      | B=[x_i1;y_i1];
      | P=[x;y];
      | Term=det([B-A,P-A]);
      | sgn=sign(Term);
      | nrm=norm(B-A);
      | d = sgn*Term/nrm; % for col. vectors
  note: update index unless heading towards last pt
  note: add the drift distance to the current distance to
      | illude the guidance system=>virtual path
  x : Inport
  y : Inport  Port=2
  index_i : Inport  Port=3
  x_dot : Inport  Port=4
  y_dot : Inport  Port=5
  alpha : Inport  Port=6
  psi : Inport  Port=7
  Add{,1,4..6} (5 alike) : Sum
  Add{2..3,7..8} (4 alike) : Sum  Inputs=+-
  Computing the intersection between the line and the circle1 : MATLAB Function  TreatAsAtomicUnit=on
  Constant{,1,4..5} (4 alike) : Constant
  Constant2 : Constant  Value=length(X_way)-1
  Constant3 : Constant  Value=length(X_way)-1
  Enabled Subsystem : Subsystem  TreatAsAtomicUnit=on
  Lookup Table : Lookup  InputValues=dist_LOS  Table=radius_LOS
  Mux : Mux  Inputs=2
  Mux1 : Mux  Inputs=2
  Product4 : Product  Inputs=**/  RndMeth=Zero
  Product5 : Product  RndMeth=Zero
  R_convrg : Constant  Value=R_convrg
  R_convrg1 : Constant  Value=1.5*R_convrg
  Relational Operator : RelationalOperator  Operator=<  OutDataTypeStr=uint(8)  RndMeth=Nearest
  Relational Operator1 : RelationalOperator  Operator===  OutDataTypeStr=boolean  RndMeth=Nearest
  Relational Operator2 : RelationalOperator  Operator=<  OutDataTypeStr=uint(8)  RndMeth=Nearest
  Relational Operator3 : RelationalOperator  Operator=~=  OutDataTypeStr=boolean  RndMeth=Nearest
  Scope{1..3,6} (4 alike) : Scope
  Sign : Signum
  Subsystem : Subsystem
  Subsystem1 : Subsystem
  norm : Fcn  Expr=sqrt(u(1)^2+u(2)^2)
  norm1 : Fcn  Expr=sqrt(u(1)^2+u(2)^2)
  x-way Lookup Table : Lookup  InputValues=INDEX  Table=X_way
  x-way Lookup Table1 : Lookup  InputValues=INDEX  Table=X_way
  x-way Lookup Table2 : Lookup  InputValues=INDEX  Table=X_way  LookUpMeth=Interpolation-Use End Values
  x-way Lookup Table3 : Lookup  InputValues=INDEX  Table=X_way  LookUpMeth=Interpolation-Use End Values
  y-way Lookup Table : Lookup  InputValues=INDEX  Table=Y_way
  y-way Lookup Table1 : Lookup  InputValues=INDEX  Table=Y_way
  y-way Lookup Table2 : Lookup  InputValues=INDEX  Table=Y_way  LookUpMeth=Interpolation-Use End Values
  y-way Lookup Table3 : Lookup  InputValues=INDEX  Table=Y_way  LookUpMeth=Interpolation-Use End Values
  index_i_update : Outport
  x_los : Outport  Port=2
  y_los : Outport  Port=3
  dist : Outport  Port=4
  Acceptance_R_Flag : Outport  Port=5
  wires:
  x/1 -> [x]
  y/1 -> [y]
  index_i/1 -> [index_i]
  [index_i] -> x-way Lookup Table/1
  [index_i] -> y-way Lookup Table/1
  x-way Lookup Table/1 -> [x_i]
  y-way Lookup Table/1 -> [y_i]
  x-way Lookup Table1/1 -> [x_i1]
  y-way Lookup Table1/1 -> [y_i1]
  [index_i] -> Add/1
  Add/1 -> x-way Lookup Table1/1
  Constant/1 -> Add/2
  [index_i] -> Add1/1
  Add1/1 -> y-way Lookup Table1/1
  Constant1/1 -> Add1/2
  [x] -> Add2/1
  [x_i1] -> Add2/2
  [y] -> Add3/1
  [y_i1] -> Add3/2
  Add2/1 -> Mux/1
  Add3/1 -> Mux/2
  Mux/1 -> norm/1
  norm/1 -> Relational Operator/1
  [index_i] -> Relational Operator1/1
  Constant2/1 -> Relational Operator1/2
  Relational Operator1/1 -> Enabled Subsystem/Enable
  R_convrg/1 -> Relational Operator/2
  Relational Operator/1 -> Product5/1
  [x] -> Enabled Subsystem/1(x)
  [y] -> Enabled Subsystem/2(y)
  Product5/1 -> Add4/1, [FLAG_cnvrg]
  Add4/1 -> [index_i_update]
  [index_i_update] -> index_i_update/1
  [index_i_update] -> x-way Lookup Table2/1
  [index_i_update] -> y-way Lookup Table2/1
  x-way Lookup Table2/1 -> [x_i_update]
  y-way Lookup Table2/1 -> [y_i_update]
  x-way Lookup Table3/1 -> [x_i1_update]
  y-way Lookup Table3/1 -> [y_i1_update]
  Add5/1 -> x-way Lookup Table3/1
  Constant4/1 -> Add5/2
  Add6/1 -> y-way Lookup Table3/1
  Constant5/1 -> Add6/2
  [index_i_update] -> Add5/1
  [index_i_update] -> Add6/1
  [x] -> Subsystem/1(x)
  [y] -> Subsystem/2(y)
  [x_i_update] -> Subsystem/3(x_i)
  [y_i_update] -> Subsystem/4(y_i)
  [x_i1_update] -> Subsystem/5(x_i1)
  [y_i1_update] -> Subsystem/6(y_i1)
  [x] -> Computing the intersection between the line and the circle1/1(x)
  [y] -> Computing the intersection between the line and the circle1/2(y)
  Subsystem/1(det) -> [det]
  [det] -> Sign/1
  [det] -> Product4/2
  Sign/1 -> [sgn_det]
  [sgn_det] -> Product4/1
  [x_i1_update] -> Subsystem1/1(x_i1)
  [x_i_update] -> Subsystem1/2("x_i ")
  [y_i1_update] -> Subsystem1/3(y_i1)
  [y_i_update] -> Subsystem1/4(y_i)
  Product4/1 -> dist/1, [dist]
  y_dot/1 -> [y_dot]
  x_dot/1 -> [x_dot]
  Subsystem1/1(norm_) -> [nrm]
  [nrm] -> Product4/3
  [R] -> Scope1/1, [Radius]
  Computing the intersection between the line and the circle1/1(x_los) -> Scope2/1, x_los/1
  Computing the intersection between the line and the circle1/2(y_los) -> Scope3/1, y_los/1
  [index_i] -> Add4/2
  [index_i] -> Relational Operator3/1
  Constant3/1 -> Relational Operator3/2
  Relational Operator3/1 -> Product5/2
  Subsystem1/2(slope_waypath) -> [slope_waypath]
  psi/1 -> [psi]
  alpha/1 -> [alpha]
  Lookup Table/1 -> [R]
  [x] -> Add7/1
  [x_i] -> Add7/2
  [y] -> Add8/1
  [y_i] -> Add8/2
  Add7/1 -> Mux1/1
  Add8/1 -> Mux1/2
  Mux1/1 -> norm1/1
  norm1/1 -> Relational Operator2/1
  R_convrg1/1 -> Relational Operator2/2
  Relational Operator2/1 -> Acceptance_R_Flag/1
  [dist] -> Scope6/1, Lookup Table/1
  [x_i_update] -> Computing the intersection between the line and the circle1/3(x_i)
  [y_i_update] -> Computing the intersection between the line and the circle1/4(y_i)
  [x_i1_update] -> Computing the intersection between the line and the circle1/5(x_i1)
  [y_i1_update] -> Computing the intersection between the line and the circle1/6(y_i1)
  [Radius] -> Computing the intersection between the line and the circle1/7(R)

== system Chapter_4_Section_3_Model/Ship_Model/Ship Dynamics with Environmental Forces and Memory Effect/Buoyancy_Forces ==
  note: Inputs
  note: V_submerged
  note: outputs
  note: gravity force(weight of the ship)
  J1 : Inport
  x : Inport  Port=2
  y : Inport  Port=3
  z : Inport  Port=4
  ksi : Inport  Port=5
  Constant28 : Constant  Value=XYZ_all
  Cross Product : Subsystem
  J1 matrix : MATLAB Function  TreatAsAtomicUnit=on
  Mux2 : Mux  Inputs=2
  Product : Product  RndMeth=Zero
  Product1 : Product  Inputs=3  RndMeth=Zero
  Product2 : Product  RndMeth=Zero
  Product3 : Product  Multiplication=Matrix(*)  RndMeth=Zero
  Product4 : Product  Multiplication=Matrix(*)  RndMeth=Zero
  Product5 : Product  Inputs=3  RndMeth=Zero
  Subsystem : Subsystem
  Sum1 : Sum  Inputs=|+|-|
  Sum2 : Sum  Inputs=|+|-|
  Unit vector opposite to the z-direction : Constant  Value=[0;0;-1]
  Unit vector opposite to the z-direction1 : Constant  Value=[0;0;1]
  "Vship_sub " : Constant  Value=Vship_sub
  "[xB,yB,zB] " : Mux  Inputs=3
  g : Constant  Value=gravity
  g1 : Constant  Value=gravity
  raw : Constant  Value=raw
  raw1 : Constant  Value=raw
  residual error in the computaion of x_buoyancy : Constant  Value=xCOB
  Gravity_Buoyancy_Force : Outport
  wires:
  [Vsub] -> Product5/3
  Cross Product/1(c) -> [Buoyancy_Moment]
  Unit vector opposite to the z-direction/1 -> Product/1
  [Buoyancy_Force] -> Product/2
  Product/1 -> Product4/2
  J1/1 -> J1 matrix/1(u), [J1]
  Mux2/1 -> Gravity_Buoyancy_Force/1
  Subsystem/1(Vsub) -> [Vsub]
  Subsystem/2(x_Buoyancy) -> Sum1/1
  residual error in the computaion of x_buoyancy/1 -> Sum1/2
  Sum1/1 -> "[xB,yB,zB] "/1
  Subsystem/3(y_Buoyancy) -> "[xB,yB,zB] "/2
  Subsystem/4(z_Buoyancy) -> "[xB,yB,zB] "/3
  "[xB,yB,zB] "/1 -> Cross Product/1(a)
  raw/1 -> Product5/1
  g/1 -> Product5/2
  [Buoyancy_Force] -> Sum2/2
  Sum2/1 -> Product2/2
  Product5/1 -> [Buoyancy_Force]
  raw1/1 -> Product1/1
  g1/1 -> Product1/2
  "Vship_sub "/1 -> Product1/3
  Product1/1 -> Sum2/1
  Product4/1 -> Cross Product/2(b)
  x/1 -> [x]
  y/1 -> [y]
  z/1 -> [z]
  [J1] -> Subsystem/1(J1)
  [x] -> Subsystem/3(x)
  [y] -> Subsystem/4(y)
  [z] -> Subsystem/5(z)
  Constant28/1 -> Subsystem/6(X1Y1Z1)
  [INV_J1] -> Product4/1
  Unit vector opposite to the z-direction1/1 -> Product2/1
  Product2/1 -> Product3/2
  [INV_J1] -> Product3/1
  Product3/1 -> [Gravity_Buoyancy_Force]
  [Gravity_Buoyancy_Force] -> Mux2/1
  [Buoyancy_Moment] -> Mux2/2
  J1 matrix/1(y) -> [INV_J1]
  [INV_J1] -> Subsystem/2(INV_J1)
  ksi/1 -> Subsystem/7(ksi)

== system Chapter_4_Section_3_Model/Ship_Model/Ship Dynamics with Environmental Forces and Memory Effect/Current Force ==
  psi : Inport
  u : Inport  Port=2
  current_angle_degree : Inport  Port=3
  velocity_current : Inport  Port=4
  Constant1 : Constant  Value=2*pi
  Constant18 : Constant  Value=360
  Constant19 : Constant  Value=raw
  Constant21 : Constant  Value=LBP
  Constant23 : Constant  Value=T
  Gain10 : Gain  Gain=pi/180
  Gain9 : Gain  Gain=180/pi
  Math Function1 : Math  Operator=mod  SaturateOnIntegerOverflow=on
  Math Function3 : Math  Operator=mod  SaturateOnIntegerOverflow=on
  Product11 : Product  RndMeth=Zero
  Subsystem4 : Subsystem
  Sum8 : Sum  Inputs=|+|-|
  Sum9 : Sum  Inputs=|+|-|
  Trigonometric Function1 : Trigonometry  Operator=cos
  F_current : Outport
  wires:
  Constant18/1 -> Math Function3/2
  current_angle_degree/1 -> Sum8/1
  Gain9/1 -> Sum8/2
  Sum8/1 -> Math Function3/1
  Math Function3/1 -> [relative_current_angle_deg]
  [relative_current_angle_deg] -> Subsystem4/1("current_encounter_angle ")
  Constant19/1 -> Subsystem4/2(density of water)
  Constant21/1 -> Subsystem4/3(LBP: length between the prependiculars)
  Constant23/1 -> Subsystem4/4("T(draft):distance from the water line to the bottom of the vessel   ")
  [relative_current_angle_deg] -> Gain10/1
  Gain10/1 -> Trigonometric Function1/1
  Trigonometric Function1/1 -> Product11/2
  Subsystem4/1(F_current) -> F_current/1
  Sum9/1 -> Subsystem4/5(Vcurrent_relative)
  Product11/1 -> Sum9/1
  u/1 -> Sum9/2
  velocity_current/1 -> Product11/1
  psi/1 -> Math Function1/1
  Constant1/1 -> Math Function1/2
  Math Function1/1 -> Gain9/1
